simulink library "ss_vec_2_angles"  (R2016b)
settings: Solver=VariableStepAuto  StartTime=0.0  StopTime=10.0  RelTol=1e-3
settings Model: Creator=taylorreynolds  LastModifiedBy=taylorreynolds

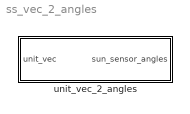
== system ss_vec_2_angles ==
  unit_vec_2_angles : Subsystem

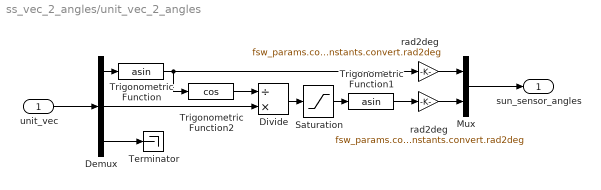
== system ss_vec_2_angles/unit_vec_2_angles ==
  unit_vec : Inport
  Demux : Demux  Outputs=3
  Divide : Product  Inputs=/*
  Mux : Mux  Inputs=2
  Saturation : Saturate  UpperLimit=1  LowerLimit=-1
  Terminator : Terminator
  Trigonometric Function : Trigonometry  Operator=asin
  Trigonometric Function1 : Trigonometry  Operator=asin
  Trigonometric Function2 : Trigonometry  Operator=cos
  rad2deg : Gain  Gain=fsw_params.constants.convert.rad2deg
  "rad2deg " : Gain  Gain=fsw_params.constants.convert.rad2deg
  sun_sensor_angles : Outport
  wires:
  unit_vec/1 -> Demux/1
  Demux/1 -> Trigonometric Function/1
  Demux/2 -> Divide/2
  Trigonometric Function/1 -> Trigonometric Function2/1, rad2deg/1
  Trigonometric Function1/1 -> "rad2deg "/1
  Mux/1 -> sun_sensor_angles/1
  Demux/3 -> Terminator/1
  rad2deg/1 -> Mux/1
  "rad2deg "/1 -> Mux/2
  Trigonometric Function2/1 -> Divide/1
  Saturation/1 -> Trigonometric Function1/1
  Divide/1 -> Saturation/1
